simulink model "IHC_Lowpass_Filter"  (R2019b)
settings: Solver=VariableStepAuto  StartTime=0.0  StopTime=testtime  RelTol=1e-3
InitFcn:
  | IHC_Lowpass_Test_Parameters
StopFcn:
  | Verify_IHC_Lowpass_Filter
values from neighbouring files (symbols this model uses):
  c1LPihc = ( C - TWOPI*Fcihc ) / ( C + TWOPI*Fcihc )    (= 0.671752219322)    [IHC_Lowpass_Test_Parameters.m]
  c2LPihc = TWOPI*Fcihc / (TWOPI*Fcihc + C)    (= 0.164123890339)    [IHC_Lowpass_Test_Parameters.m]
  Fs = 48e3    (= 48000)    [IHC_Lowpass_Test_Parameters.m]
  gainihc = 1.0    (= 1)    [IHC_Lowpass_Test_Parameters.m]
  IHCLPcoeffs = [  gainihc*c2LPihc gainihc*c2LPihc 0 1 -c1LPihc 0 ... (first row only)    [IHC_Lowpass_Test_Parameters.m]
undefined symbols (not defined in the file or in its folder): dfilt
libraries: dsparch4 x4, dspsrcs4 x2
settings Model: Creator=mblun  LastModifiedBy=t96f346
settings OptimizationCC: BlockReduction=off  ConditionallyExecuteInputs=off  DefaultParameterBehavior=Inlined
settings DebuggingCC: AlgebraicLoopMsg=error
settings HardwareCC: ProdBitPerPointer=32  ProdBitPerSizeT=32  ProdBitPerPtrDiffT=32  ProdLargestAtomicFloat=None  ProdIntDivRoundTo=Undefined  ProdEndianess=Unspecified  ProdWordSize=32  ProdHWDeviceType=ASIC/FPGA->ASIC/FPGA  TargetBitPerPointer=64  TargetBitPerSizeT=64  TargetBitPerPtrDiffT=64  TargetLongLongMode=on  TargetIntDivRoundTo=Zero  TargetEndianess=LittleEndian  TargetWordSize=64  TargetHWDeviceType=Custom Processor->MATLAB Host Computer  ProdEqTarget=off
settings SFSimCC: CustomCodeUndefinedFunction=UseInterfaceOnly

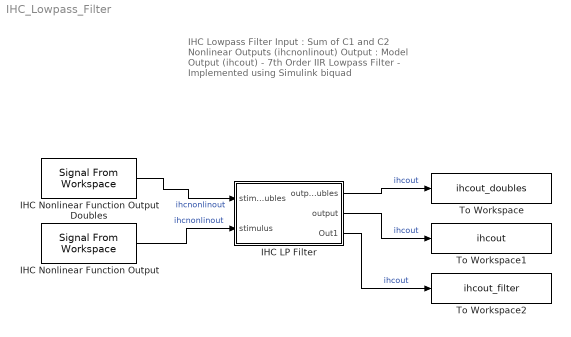
== system IHC_Lowpass_Filter ==
  note: IHC Lowpass Filter
      |
      | Input : Sum of C1 and C2 Nonlinear Outputs (ihcnonlinout)
      |
      | Output : Model Output (ihcout)
      |
      | - 7th Order IIR Lowpass Filter
      |
      | - Implemented using Simulink biquad
  IHC LP Filter : Subsystem
  IHC Nonlinear Function Output : dspsrcs4/Signal From Workspace  X=RxSignal  Ts=1/Fs  nsamps=1  OutputAfterFinalValue=Setting to zero  ignoreOrWarnInputAndFrameLengths=off  OutputFrames=off
  IHC Nonlinear Function Output Doubles : dspsrcs4/Signal From Workspace  X=RxSignal_doubles  Ts=1/Fs  nsamps=1  OutputAfterFinalValue=Setting to zero  ignoreOrWarnInputAndFrameLengths=off  OutputFrames=off
  To Workspace : ToWorkspace  VariableName=ihcout_doubles  SampleTime=-1
      settings: Save2DSignal=2-D array (concatenate along first dimension)
  To Workspace1 : ToWorkspace  VariableName=ihcout  SampleTime=-1
      settings: Save2DSignal=2-D array (concatenate along first dimension)
  To Workspace2 : ToWorkspace  VariableName=ihcout_filter  SampleTime=-1
      settings: Save2DSignal=2-D array (concatenate along first dimension)
  wires:
  IHC Nonlinear Function Output Doubles/1 -> IHC LP Filter/1(stimulus_doubles)  "ihcnonlinout"
  IHC LP Filter/2(output) -> To Workspace1/1  "ihcout"
  IHC Nonlinear Function Output/1 -> IHC LP Filter/2(stimulus)  "ihcnonlinout"
  IHC LP Filter/1(output_doubles) -> To Workspace/1  "ihcout"
  IHC LP Filter/3(Out1) -> To Workspace2/1  "ihcout"

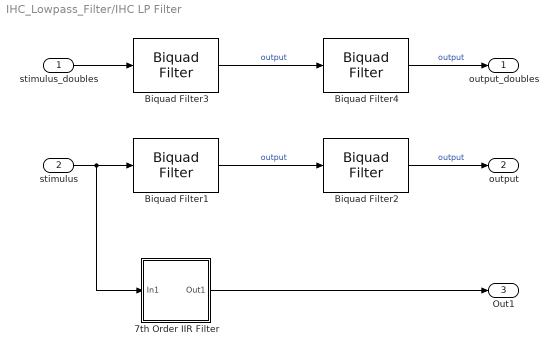
== system IHC_Lowpass_Filter/IHC LP Filter ==
  stimulus_doubles : Inport
  stimulus : Inport  Port=2
  7th Order IIR Filter : Subsystem
  Biquad Filter1 : dsparch4/Biquad Filter  FilterSource=Dialog parameters  CoeffSource=Specify via dialog  FilterObject=dfilt.df2tsos([1 0.3 0.4],[1 0.1 0.2])  IIRFiltStruct=Direct form I  BiQuadCoeffs=[gainihc*c2LPihc gainihc*c2LPihc 0 1 -c1LPihc 0; c2LPihc c2LPihc 0 1 -c1LPihc 0; c2LPihc c2LPihc 0 1 -c1LPihc 0;c2LPihc c2LPihc 0 1 -c1LPihc 0]  ScaleValues=1  IC=0  ICnum=0  ICden=0  a0Flag=Warning  optimizeScaleValues=on  ScaleValueMode=Specify via input port (g)  roundingMode=Floor  overflowMode=on  scaleValueFracLength=14  denProdOutputFracLength=30  denAccumFracLength=30  secondMemoryFracLength=15
      settings: SourceProductName=DSP System Toolbox
  Biquad Filter2 : dsparch4/Biquad Filter  FilterSource=Dialog parameters  CoeffSource=Specify via dialog  FilterObject=dfilt.df2tsos([1 0.3 0.4],[1 0.1 0.2])  IIRFiltStruct=Direct form I  BiQuadCoeffs=[c2LPihc c2LPihc 0 1 -c1LPihc 0; c2LPihc c2LPihc 0 1 -c1LPihc 0; c2LPihc c2LPihc 0 1 -c1LPihc 0]  ScaleValues=1  IC=0  ICnum=0  ICden=0  a0Flag=Warning  optimizeScaleValues=on  ScaleValueMode=Specify via input port (g)  roundingMode=Floor  overflowMode=on  scaleValueFracLength=14  denProdOutputFracLength=30  denAccumFracLength=30  secondMemoryFracLength=15
      settings: SourceProductName=DSP System Toolbox
  Biquad Filter3 : dsparch4/Biquad Filter  FilterSource=Dialog parameters  CoeffSource=Specify via dialog  FilterObject=dfilt.df2tsos([1 0.3 0.4],[1 0.1 0.2])  IIRFiltStruct=Direct form I  BiQuadCoeffs=[gainihc*c2LPihc gainihc*c2LPihc 0 1 -c1LPihc 0; c2LPihc c2LPihc 0 1 -c1LPihc 0; c2LPihc c2LPihc 0 1 -c1LPihc 0;c2LPihc c2LPihc 0 1 -c1LPihc 0]  ScaleValues=1  IC=0  ICnum=0  ICden=0  a0Flag=Warning  optimizeScaleValues=on  ScaleValueMode=Specify via input port (g)  roundingMode=Floor  overflowMode=on  scaleValueFracLength=14  denProdOutputFracLength=30  denAccumFracLength=30  secondMemoryFracLength=15
      settings: SourceProductName=DSP System Toolbox
  Biquad Filter4 : dsparch4/Biquad Filter  FilterSource=Dialog parameters  CoeffSource=Specify via dialog  FilterObject=dfilt.df2tsos([1 0.3 0.4],[1 0.1 0.2])  IIRFiltStruct=Direct form I  BiQuadCoeffs=[c2LPihc c2LPihc 0 1 -c1LPihc 0; c2LPihc c2LPihc 0 1 -c1LPihc 0; c2LPihc c2LPihc 0 1 -c1LPihc 0]  ScaleValues=1  IC=0  ICnum=0  ICden=0  a0Flag=Warning  optimizeScaleValues=on  ScaleValueMode=Specify via input port (g)  roundingMode=Floor  overflowMode=on  scaleValueFracLength=14  denProdOutputFracLength=30  denAccumFracLength=30  secondMemoryFracLength=15
      settings: SourceProductName=DSP System Toolbox
  output_doubles : Outport  VectorParamsAs1DForOutWhenUnconnected=off
  output : Outport  Port=2  VectorParamsAs1DForOutWhenUnconnected=off
  Out1 : Outport  Port=3  VectorParamsAs1DForOutWhenUnconnected=off
  wires:
  Biquad Filter1/1 -> Biquad Filter2/1  "output"
  Biquad Filter2/1 -> output/1  "output"
  stimulus_doubles/1 -> Biquad Filter3/1
  Biquad Filter3/1 -> Biquad Filter4/1  "output"
  Biquad Filter4/1 -> output_doubles/1  "output"
  stimulus/1 -> 7th Order IIR Filter/1(In1), Biquad Filter1/1
  7th Order IIR Filter/1(Out1) -> Out1/1

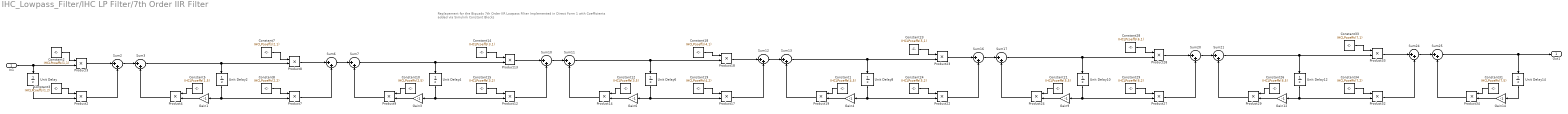
== system IHC_Lowpass_Filter/IHC LP Filter/7th Order IIR Filter ==
  note: Replacement for the Biquads
      | 7th Order IIR Lowpass Filter Implemented in Direct Form 1 with Coefficients added via Simulink Constant Blocks
  In1 : Inport  OutDataTypeStr=single
  Constant1 : Constant  Value=IHCLPcoeffs(4,5)  OutDataTypeStr=single  SampleTime=-1
  Constant10 : Constant  Value=IHCLPcoeffs(2,5)  OutDataTypeStr=single  SampleTime=-1
  Constant12 : Constant  Value=IHCLPcoeffs(3,5)  OutDataTypeStr=single  SampleTime=-1
  Constant14 : Constant  Value=IHCLPcoeffs(3,1)  OutDataTypeStr=single  SampleTime=-1
  Constant15 : Constant  Value=IHCLPcoeffs(3,2)  OutDataTypeStr=single  SampleTime=-1
  Constant18 : Constant  Value=IHCLPcoeffs(4,1)  OutDataTypeStr=single  SampleTime=-1
  Constant19 : Constant  Value=IHCLPcoeffs(4,2)  OutDataTypeStr=single  SampleTime=-1
  Constant2 : Constant  Value=IHCLPcoeffs(1,1)  OutDataTypeStr=single  SampleTime=-1
  Constant21 : Constant  Value=IHCLPcoeffs(5,5)  OutDataTypeStr=single  SampleTime=-1
  Constant23 : Constant  Value=IHCLPcoeffs(5,1)  OutDataTypeStr=single  SampleTime=-1
  Constant24 : Constant  Value=IHCLPcoeffs(5,2)  OutDataTypeStr=single  SampleTime=-1
  Constant26 : Constant  Value=IHCLPcoeffs(6,5)  OutDataTypeStr=single  SampleTime=-1
  Constant28 : Constant  Value=IHCLPcoeffs(6,1)  OutDataTypeStr=single  SampleTime=-1
  Constant29 : Constant  Value=IHCLPcoeffs(6,2)  OutDataTypeStr=single  SampleTime=-1
  Constant3 : Constant  Value=IHCLPcoeffs(1,2)  OutDataTypeStr=single  SampleTime=-1
  Constant31 : Constant  Value=IHCLPcoeffs(7,5)  OutDataTypeStr=single  SampleTime=-1
  Constant33 : Constant  Value=IHCLPcoeffs(7,1)  OutDataTypeStr=single  SampleTime=-1
  Constant34 : Constant  Value=IHCLPcoeffs(7,2)  OutDataTypeStr=single  SampleTime=-1
  Constant5 : Constant  Value=IHCLPcoeffs(1,5)  OutDataTypeStr=single  SampleTime=-1
  Constant7 : Constant  Value=IHCLPcoeffs(2,1)  OutDataTypeStr=single  SampleTime=-1
  Constant8 : Constant  Value=IHCLPcoeffs(2,2)  OutDataTypeStr=single  SampleTime=-1
  Gain{1,3..4,6,9,12,14} (7 alike) : Gain  Gain=-1
  Product{2..4,7..9,12..14,17..19,22..24,27..29,32..34} (21 alike) : Product
  Sum{2..3,6..7,10..13,16..17,20..21,24..25} (14 alike) : Sum  Inputs=|++
  Unit Delay{,2,4,6,8,10,12,14} (8 alike) : UnitDelay  SampleTime=-1  HasFrameUpgradeWarning=on
  Out1 : Outport  OutDataTypeStr=single
  wires:
  Product7/1 -> Sum6/2
  Product2/1 -> Sum2/2
  Sum6/1 -> Sum7/1
  Sum2/1 -> Sum3/1
  Constant8/1 -> Product7/1
  Product19/1 -> Sum13/2
  Constant10/1 -> Product9/1
  Constant5/1 -> Product4/1
  Product9/1 -> Sum7/2
  Constant18/1 -> Product18/1
  Constant12/1 -> Product14/1
  Constant14/1 -> Product13/1
  Sum17/1 -> Unit Delay10/1, Product28/2
  Product13/1 -> Sum10/1
  Product17/1 -> Sum12/2
  Gain3/1 -> Product9/2
  Unit Delay/1 -> Product2/2
  Unit Delay8/1 -> Product22/2, Gain4/1
  Product22/1 -> Sum16/2
  Sum3/1 -> Unit Delay2/1, Product8/2
  Product23/1 -> Sum16/1
  Product3/1 -> Sum2/1
  Constant3/1 -> Product2/1
  Constant21/1 -> Product24/1
  Unit Delay2/1 -> Product7/2, Gain1/1
  Constant19/1 -> Product17/1
  Sum16/1 -> Sum17/1
  Constant15/1 -> Product12/1
  Product18/1 -> Sum12/1
  Sum11/1 -> Unit Delay6/1, Product18/2
  Product4/1 -> Sum3/2
  Unit Delay6/1 -> Product17/2, Gain6/1
  Unit Delay10/1 -> Product27/2, Gain9/1
  Gain9/1 -> Product24/2
  Sum10/1 -> Sum11/1
  Gain4/1 -> Product19/2
  Product14/1 -> Sum11/2
  Gain1/1 -> Product4/2
  Product12/1 -> Sum10/2
  Sum7/1 -> Unit Delay4/1, Product13/2
  Sum13/1 -> Unit Delay8/1, Product23/2
  Gain6/1 -> Product14/2
  Constant24/1 -> Product22/1
  Product24/1 -> Sum17/2
  Unit Delay4/1 -> Product12/2, Gain3/1
  Constant1/1 -> Product19/1
  Product8/1 -> Sum6/1
  In1/1 -> Product3/2, Unit Delay/1
  Constant7/1 -> Product8/1
  Constant2/1 -> Product3/1
  Constant23/1 -> Product23/1
  Sum12/1 -> Sum13/1
  Constant28/1 -> Product28/1
  Constant29/1 -> Product27/1
  Unit Delay12/1 -> Product32/2, Gain12/1
  Product28/1 -> Sum20/1
  Product27/1 -> Sum20/2
  Sum21/1 -> Unit Delay12/1, Product33/2
  Gain12/1 -> Product29/2
  Sum20/1 -> Sum21/1
  Product29/1 -> Sum21/2
  Constant26/1 -> Product29/1
  Constant33/1 -> Product33/1
  Constant34/1 -> Product32/1
  Unit Delay14/1 -> Gain14/1
  Product33/1 -> Sum24/1
  Product32/1 -> Sum24/2
  Sum25/1 -> Out1/1, Unit Delay14/1
  Gain14/1 -> Product34/2
  Sum24/1 -> Sum25/1
  Product34/1 -> Sum25/2
  Constant31/1 -> Product34/1
